simulink model "Lab04"  (R2018a)
settings: Solver=VariableStepAuto  StartTime=0.0  StopTime=10.0  RelTol=1e-3
libraries: simulink_extras x1
settings Model: Creator=Wellter Sozin  LastModifiedBy=Wellter Sozin

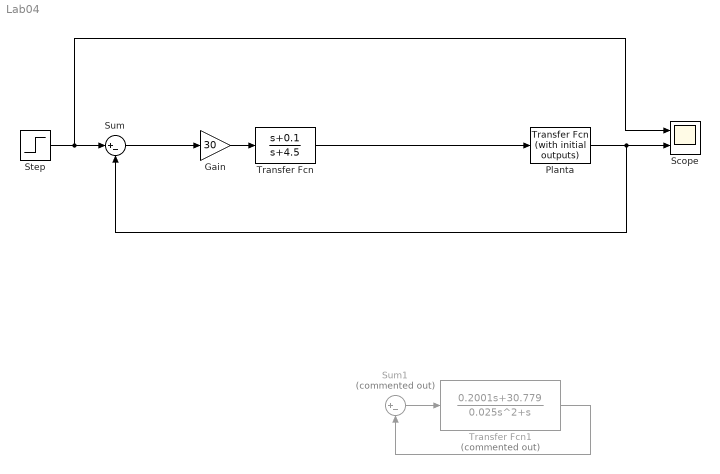
== system Lab04 ==
  Gain : Gain  Gain=30
  Planta : simulink_extras/Additional Linear/Transfer Fcn (with initial outputs)  N=[0.21]  D=[1 0 0]  Y0=.2  U0=0
  Scope : Scope  NumInputPorts=2
  Step : Step  After=0.15  SampleTime=0
  Sum : Sum  Inputs=|+-
  Sum1 : Sum  Commented=on  Inputs=|+-
  Transfer Fcn : TransferFcn  Numerator=[1 0.1]  Denominator=[1 4.5]
  Transfer Fcn1 : TransferFcn  Commented=on  Numerator=[0.2001 30.779]  Denominator=[0.025 1 0]
  wires:
  Gain/1 -> Transfer Fcn/1
  Sum/1 -> Gain/1
  Planta/1 -> Sum/2, Scope/2
  Step/1 -> Scope/1, Sum/1
  Sum1/1 -> Transfer Fcn1/1
  Transfer Fcn1/1 -> Sum1/2
  Transfer Fcn/1 -> Planta/1
